simulink model "sampleModel1501"  (R2023a)
settings: Solver=VariableStepAuto  StartTime=0.0  StopTime=10.0  RelTol=1e-3
libraries: hdlsllib x5, simulink x1
settings Model: Creator=user1  LastModifiedBy=user1

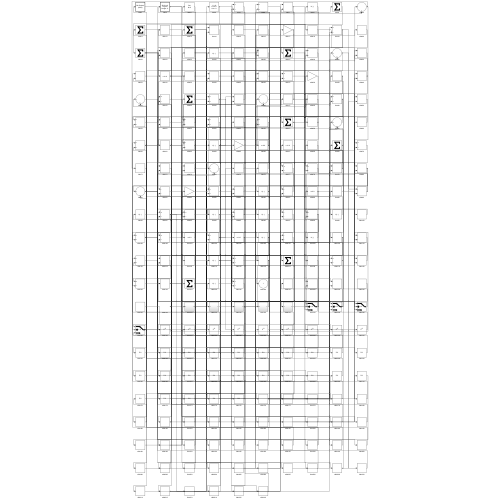
[thumbnail: Simulink's stored preview of the top-level diagram]
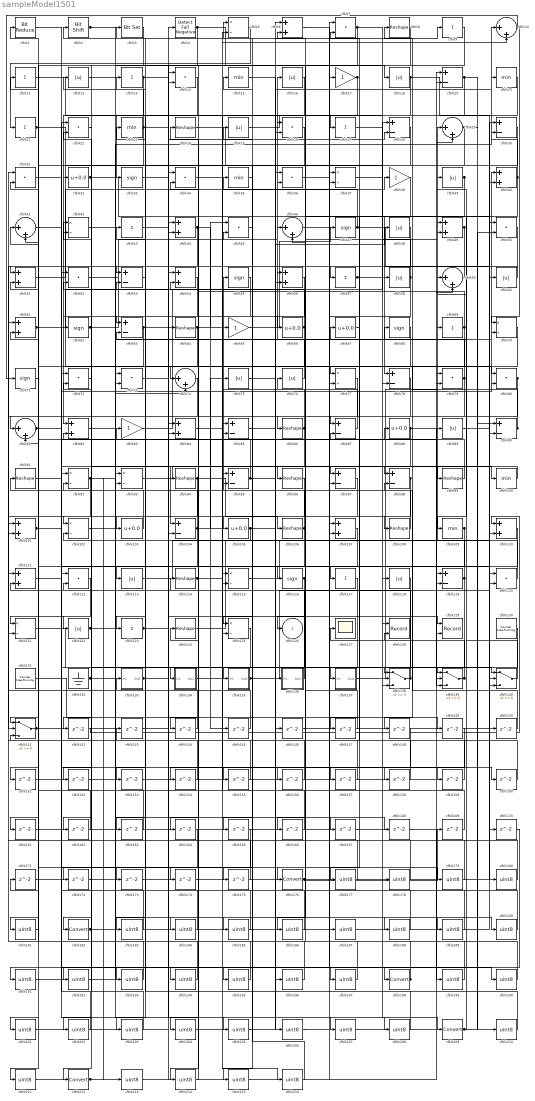
== system sampleModel1501 ==
  cfblk1 : hdlsllib/Logic and Bit Operations/Bit Reduce  mode=AND
  cfblk{10,29,41,46,59,74,81} (7 alike) : Sum  Inputs=|++
  cfblk{15,20,23,35,100,109} (6 alike) : MinMax
  cfblk{6,40,44,49,51,54,56,61,82,84,101,107,110..111} (14 alike) : Sum
  cfblk{5,37,42,70,77,92..93,102,115,121,125} (11 alike) : Product  Inputs=*/  RndMeth=Zero  SaturateOnIntegerOverflow=on
  cfblk{32,66..67,88,103,105} (6 alike) : Bias  Bias=0.0  SaturateOnIntegerOverflow=off
  cfblk{19,28,30,53,63,78,85,87,90,95,97..98,104,119} (14 alike) : Sum  Inputs=+-
  cfblk{8,24,64,86,91,94,96,99,106,108,114,124} (12 alike) : Reshape
  cfblk{9,11,13,21,27,43,57,69,117,123} (10 alike) : Sum  Inputs=+
  cfblk{7,14,22,26,31,34,36,45,50,52,72..73,79..80,112,120} (16 alike) : DotProduct  OutDataTypeStr=Inherit: Inherit via internal rule
  cfblk{12,16,18,25,39,48,58,60,75..76,89,113,118,122} (14 alike) : Abs  SaturateOnIntegerOverflow=off
  cfblk{33,47,55,62,68,71,116} (7 alike) : Signum
  cfblk127 : Scope
  cfblk128 : Record  FileSettingsInternal="{\"entries\":[{\"content\":{\"excelSettings\":{\"content\":{},\"type\":\"Streamout.ExcelSettings\"}},\"type\":\"Streamout.FileSettingStorage\",\"uuid\":\"\"}],\"packageUris\":[\"http:\\/\\/schema.mathworks.com\\/mf0\\/streamout_blocks\\/R2020a\"],\"version\":\"1.0\"}"  Layout=[1 1]  SignalsInternal="{\"entries\":[{\"content\":{\"signals\":[{\"content\":{\"blockPath\":[],\"dimensions\":[1],\"domain\":\"\",\"lineColor\":\"#a2142f\",\"plots\":[1],\"port\":1,\"signalID\":1280,\"signalName\":\"XY Graph:1\"},\"type\":\"RecordBlkView.Signal\",\"uuid\":\"\"},{\"content\":{\"blockPath\":[],\"dimensions\":[1],\"domain\":\"\",\"lineColor\":\"#139fff\",\"plots\":[1],\"port\":2,\"signalID\":1283,\"signalName\":\"XY Graph:2\"},\"type\":\"RecordBlkView.Signal\",\"uuid\":\"\"}]},\"type\":\"RecordBlkView.InputSignals\",\"uuid\":\"\"}],\"packageUris\":[\"http:\\/\\/schema.mathworks.com\\/mf0\\/streamout_blocks\\/R2020a\"],\"version\":\"1.0\"}"  VisualizationBindings="{\"xyplotplugin\":{\"info\":[{\"series\":[{\"bindingParametersList\":[{\"parameter\":\"X-Axis\",\"signalID\":1280,\"signalName\":\"XY Graph:1\"},{\"parameter\":\"Y-Axis\",\"signalID\":1283,\"signalName\":\"XY Graph:2\"}],\"seriesID\":5430}],\"subplotID\":1}]}}"  CompatibilityTag=XY  st=-1
  cfblk129 : Record  FileSettingsInternal="{\"entries\":[{\"content\":{\"excelSettings\":{\"content\":{},\"type\":\"Streamout.ExcelSettings\"}},\"type\":\"Streamout.FileSettingStorage\",\"uuid\":\"\"}],\"packageUris\":[\"http:\\/\\/schema.mathworks.com\\/mf0\\/streamout_blocks\\/R2020a\"],\"version\":\"1.0\"}"  Layout=[1 1]  SignalsInternal="{\"entries\":[{\"content\":{\"signals\":[{\"content\":{\"blockPath\":[],\"dimensions\":[1],\"domain\":\"\",\"lineColor\":\"#a2142f\",\"plots\":[1],\"port\":1,\"signalID\":1288,\"signalName\":\"XY Graph:1\"},\"type\":\"RecordBlkView.Signal\",\"uuid\":\"\"},{\"content\":{\"blockPath\":[],\"dimensions\":[1],\"domain\":\"\",\"lineColor\":\"#139fff\",\"plots\":[1],\"port\":2,\"signalID\":1291,\"signalName\":\"XY Graph:2\"},\"type\":\"RecordBlkView.Signal\",\"uuid\":\"\"}]},\"type\":\"RecordBlkView.InputSignals\",\"uuid\":\"\"}],\"packageUris\":[\"http:\\/\\/schema.mathworks.com\\/mf0\\/streamout_blocks\\/R2020a\"],\"version\":\"1.0\"}"  VisualizationBindings="{\"xyplotplugin\":{\"info\":[{\"series\":[{\"bindingParametersList\":[{\"parameter\":\"X-Axis\",\"signalID\":1288,\"signalName\":\"XY Graph:1\"},{\"parameter\":\"Y-Axis\",\"signalID\":1291,\"signalName\":\"XY Graph:2\"}],\"seriesID\":12827}],\"subplotID\":1}]}}"  CompatibilityTag=XY  st=-1
  cfblk130 : hdlsllib/Sources/Counter Free-Running  NumBits=16  tsamp=-1
  cfblk131 : hdlsllib/Sources/Counter Free-Running  NumBits=16  tsamp=-1
  cfblk132 : Ground
  cfblk133 : Subsystem
      settings: LibrarySourceBlock=|
      | hdlsllib/Ports &
      | Subsystems/Subsystem
  cfblk134 : Subsystem
      settings: LibrarySourceBlock=|
      | hdlsllib/Ports &
      | Subsystems/Subsystem
  cfblk135 : Subsystem
      settings: LibrarySourceBlock=|
      | hdlsllib/Ports &
      | Subsystems/Subsystem
  cfblk136 : Subsystem
      settings: LibrarySourceBlock=|
      | hdlsllib/Ports &
      | Subsystems/Subsystem
  cfblk137 : Subsystem
      settings: LibrarySourceBlock=|
      | hdlsllib/Ports &
      | Subsystems/Subsystem
  cfblk{138..141} (4 alike) : Switch  SaturateOnIntegerOverflow=off  InputSameDT=off
  cfblk{142..175} (34 alike) : Delay  SampleTime=1
  cfblk{17,38,65,83} (4 alike) : Gain
  cfblk{176,182,198,209,212} (5 alike) : DataTypeConversion  SaturateOnIntegerOverflow=off  RndMeth=Floor
  cfblk{177..181,183..197,199..208,210..211,213..216} (36 alike) : DataTypeConversion  OutDataTypeStr=uint8  SaturateOnIntegerOverflow=off  RndMeth=Floor
  cfblk2 : hdlsllib/Logic and Bit Operations/Bit Shift  mode=Shift Left Logical  N=0
  cfblk3 : simulink/Logic and Bit Operations/Bit Set  iBit=0
      settings: LibrarySourceBlock=|
      | hdlsllib/Logic and Bit
      | Operations/Bit Set
  cfblk4 : hdlsllib/Logic and Bit Operations/Detect Fall Negative  vinit=0  OutDataTypeStr=boolean
  cfblk126 : Outport  VectorParamsAs1DForOutWhenUnconnected=off
  wires:
  cfblk96/1 -> cfblk105/1
  cfblk65/1 -> cfblk47/1
  cfblk92/1 -> cfblk85/2, cfblk121/1, cfblk74/2, cfblk213/1
  cfblk13/1 -> cfblk82/1, cfblk129/1, cfblk80/1
  cfblk8/1 -> cfblk134/1(In1)
  cfblk94/1 -> cfblk106/1, cfblk101/2
  cfblk60/1 -> cfblk51/1
  cfblk64/1 -> cfblk103/1, cfblk45/1, cfblk139/3, cfblk10/2
  cfblk106/1 -> cfblk125/1, cfblk11/1, cfblk151/1
  cfblk17/1 -> cfblk95/2, cfblk142/1
  cfblk51/1 -> cfblk38/1
  cfblk76/1 -> cfblk16/1
  cfblk136/1(Out1) -> cfblk91/1
  cfblk79/1 -> cfblk8/1, cfblk23/1, cfblk166/1
  cfblk122/1 -> cfblk188/1, cfblk208/1
  cfblk93/1 -> cfblk100/1
  cfblk46/1 -> cfblk17/1
  cfblk40/1 -> cfblk10/1, cfblk109/1
  cfblk62/1 -> cfblk46/1, cfblk138/1
  cfblk25/1 -> cfblk27/1
  cfblk115/1 -> cfblk29/1
  cfblk39/1 -> cfblk78/1, cfblk97/1
  cfblk6/1 -> cfblk198/1
  cfblk19/1 -> cfblk90/1, cfblk97/2, cfblk183/1
  cfblk30/1 -> cfblk113/1
  cfblk32/1 -> cfblk110/2, cfblk184/1
  cfblk20/1 -> cfblk86/1
  cfblk137/1(Out1) -> cfblk49/1
  cfblk123/1 -> cfblk87/2, cfblk159/1
  cfblk10/1 -> cfblk71/1, cfblk70/1
  cfblk108/1 -> cfblk55/1
  cfblk59/1 -> cfblk57/1
  cfblk5/1 -> cfblk21/1
  cfblk52/1 -> cfblk20/1
  cfblk124/1 -> cfblk30/1
  cfblk21/1 -> cfblk128/1, cfblk136/1(In1), cfblk200/1
  cfblk3/1 -> cfblk32/1
  cfblk90/1 -> cfblk40/1, cfblk68/1
  cfblk97/1 -> cfblk102/1
  cfblk88/1 -> cfblk104/1, cfblk140/3
  cfblk86/1 -> cfblk76/1, cfblk122/1
  cfblk99/1 -> cfblk3/1
  cfblk83/1 -> cfblk28/1
  cfblk66/1 -> cfblk63/1, cfblk42/2, cfblk74/1
  cfblk87/1 -> cfblk65/1
  cfblk100/1 -> cfblk98/1
  cfblk98/1 -> cfblk108/1, cfblk126/1
  cfblk119/1 -> cfblk92/2, cfblk186/1
  cfblk50/1 -> cfblk53/1
  cfblk61/1 -> cfblk56/1, cfblk139/2
  cfblk63/1 -> cfblk81/1, cfblk45/2
  cfblk16/1 -> cfblk33/1
  cfblk38/1 -> cfblk96/1
  cfblk53/1 -> cfblk13/1
  cfblk75/1 -> cfblk9/1
  cfblk141/1 -> cfblk64/1, cfblk205/1
  cfblk22/1 -> cfblk182/1
  cfblk24/1 -> cfblk118/1
  cfblk56/1 -> cfblk66/1
  cfblk114/1 -> cfblk26/1, cfblk168/1
  cfblk55/1 -> cfblk84/2
  cfblk103/1 -> cfblk51/2
  cfblk9/1 -> cfblk116/1
  cfblk11/1 -> cfblk58/1
  cfblk54/1 -> cfblk212/1
  cfblk33/1 -> cfblk4/1
  cfblk80/1 -> cfblk87/1, cfblk121/2
  cfblk47/1 -> cfblk25/1, cfblk90/2
  cfblk130/1 -> cfblk135/1(In1)
  cfblk7/1 -> cfblk99/1, cfblk141/1
  cfblk138/1 -> cfblk128/2, cfblk114/1
  cfblk44/1 -> cfblk141/2, cfblk145/1
  cfblk4/1 -> cfblk78/2, cfblk104/2
  cfblk109/1 -> cfblk125/2, cfblk162/1
  cfblk45/1 -> cfblk5/1
  cfblk134/1(Out1) -> cfblk88/1
  cfblk132/1 -> cfblk82/2, cfblk30/2
  cfblk81/1 -> cfblk115/2, cfblk140/2, cfblk80/2
  cfblk139/1 -> cfblk127/1, cfblk39/1
  cfblk58/1 -> cfblk2/1, cfblk77/2
  cfblk49/1 -> cfblk173/1, cfblk174/1
  cfblk42/1 -> cfblk94/1
  cfblk69/1 -> cfblk24/1, cfblk77/1
  cfblk23/1 -> cfblk12/1, cfblk138/2, cfblk120/2, cfblk181/1
  cfblk105/1 -> cfblk102/2, cfblk70/2
  cfblk133/1(Out1) -> cfblk89/1, cfblk28/2
  cfblk14/1 -> cfblk62/1
  cfblk37/1 -> cfblk209/1
  cfblk140/1 -> cfblk69/1
  cfblk18/1 -> cfblk120/1, cfblk26/2
  cfblk95/1 -> cfblk61/2, cfblk48/1
  cfblk121/1 -> cfblk139/1
  cfblk31/1 -> cfblk176/1
  cfblk116/1 -> cfblk164/1, cfblk165/1
  cfblk2/1 -> cfblk140/1, cfblk18/1
  cfblk29/1 -> cfblk138/3, cfblk210/1
  cfblk101/1 -> cfblk117/1, cfblk157/1
  cfblk91/1 -> cfblk85/1
  cfblk1/1 -> cfblk93/2
  cfblk120/1 -> cfblk34/2
  cfblk135/1(Out1) -> cfblk60/1, cfblk189/1
  cfblk104/1 -> cfblk42/1, cfblk123/1, cfblk75/1, cfblk158/1
  cfblk113/1 -> cfblk19/2
  cfblk57/1 -> cfblk137/1(In1), cfblk49/2
  cfblk102/1 -> cfblk67/1
  cfblk142/1 -> cfblk110/1
  cfblk28/1 -> cfblk144/1
  cfblk144/1 -> cfblk1/1
  cfblk145/1 -> cfblk61/1
  cfblk146/1 -> cfblk50/1
  cfblk67/1 -> cfblk147/1
  cfblk147/1 -> cfblk46/2
  cfblk70/1 -> cfblk148/1
  cfblk85/1 -> cfblk149/1
  cfblk150/1 -> cfblk98/2
  cfblk151/1 -> cfblk19/1
  cfblk125/1 -> cfblk152/1
  cfblk152/1 -> cfblk44/1
  cfblk118/1 -> cfblk153/1
  cfblk153/1 -> cfblk5/2
  cfblk77/1 -> cfblk154/1
  cfblk154/1 -> cfblk63/2
  cfblk26/1 -> cfblk155/1
  cfblk155/1 -> cfblk93/1
  cfblk117/1 -> cfblk156/1
  cfblk156/1 -> cfblk101/1
  cfblk157/1 -> cfblk53/2
  cfblk158/1 -> cfblk7/2
  cfblk159/1 -> cfblk92/1
  cfblk27/1 -> cfblk160/1
  cfblk160/1 -> cfblk115/1
  cfblk71/1 -> cfblk161/1
  cfblk161/1 -> cfblk29/2
  cfblk162/1 -> cfblk81/2
  cfblk68/1 -> cfblk163/1
  cfblk163/1 -> cfblk52/1
  cfblk166/1 -> cfblk95/1
  cfblk12/1 -> cfblk167/1
  cfblk169/1 -> cfblk141/3
  cfblk171/1 -> cfblk119/2
  cfblk74/1 -> cfblk172/1
  cfblk172/1 -> cfblk56/2
  cfblk173/1 -> cfblk14/2
  cfblk174/1 -> cfblk59/2
  cfblk48/1 -> cfblk175/1
  cfblk175/1 -> cfblk84/1
  cfblk176/1 -> cfblk169/1, cfblk40/2, cfblk79/2
  cfblk78/1 -> cfblk177/1
  cfblk177/1 -> cfblk31/1
  cfblk167/1 -> cfblk178/1
  cfblk178/1 -> cfblk31/2
  cfblk41/1 -> cfblk179/1
  cfblk179/1 -> cfblk83/1
  cfblk89/1 -> cfblk180/1
  cfblk180/1 -> cfblk41/1
  cfblk181/1 -> cfblk41/2
  cfblk182/1 -> cfblk150/1, cfblk52/2
  cfblk183/1 -> cfblk22/1
  cfblk184/1 -> cfblk22/2
  cfblk143/1 -> cfblk185/1
  cfblk185/1 -> cfblk72/2
  cfblk186/1 -> cfblk143/1
  cfblk36/1 -> cfblk187/1
  cfblk187/1 -> cfblk170/1
  cfblk188/1 -> cfblk36/1
  cfblk189/1 -> cfblk36/2
  cfblk73/1 -> cfblk190/1
  cfblk190/1 -> cfblk119/1
  cfblk170/1 -> cfblk191/1
  cfblk191/1 -> cfblk73/1
  cfblk72/1 -> cfblk192/1
  cfblk192/1 -> cfblk73/2
  cfblk111/1 -> cfblk193/1
  cfblk193/1 -> cfblk72/1
  cfblk149/1 -> cfblk194/1
  cfblk194/1 -> cfblk111/1
  cfblk82/1 -> cfblk195/1
  cfblk195/1 -> cfblk111/2
  cfblk15/1 -> cfblk196/1
  cfblk196/1 -> cfblk133/1(In1)
  cfblk34/1 -> cfblk197/1
  cfblk197/1 -> cfblk15/1
  cfblk198/1 -> cfblk171/1, cfblk124/1
  cfblk168/1 -> cfblk199/1
  cfblk199/1 -> cfblk6/1
  cfblk200/1 -> cfblk6/2
  cfblk112/1 -> cfblk201/1
  cfblk201/1 -> cfblk14/1
  cfblk110/1 -> cfblk202/1
  cfblk202/1 -> cfblk112/1
  cfblk164/1 -> cfblk203/1
  cfblk203/1 -> cfblk112/2
  cfblk107/1 -> cfblk204/1
  cfblk204/1 -> cfblk146/1
  cfblk205/1 -> cfblk107/1
  cfblk131/1 -> cfblk206/1
  cfblk206/1 -> cfblk107/2
  cfblk43/1 -> cfblk207/1
  cfblk207/1 -> cfblk79/1
  cfblk208/1 -> cfblk43/1
  cfblk209/1 -> cfblk59/1, cfblk50/2
  cfblk210/1 -> cfblk37/1
  cfblk165/1 -> cfblk211/1
  cfblk211/1 -> cfblk37/2
  cfblk212/1 -> cfblk129/2, cfblk44/2, cfblk34/1
  cfblk213/1 -> cfblk54/1
  cfblk148/1 -> cfblk214/1
  cfblk214/1 -> cfblk54/2
  cfblk35/1 -> cfblk215/1
  cfblk215/1 -> cfblk7/1
  cfblk84/1 -> cfblk216/1
  cfblk216/1 -> cfblk35/1

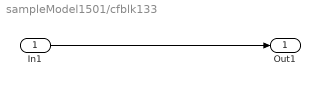
== system sampleModel1501/cfblk133 ==
  In1 : Inport
  Out1 : Outport
  wires:
  In1/1 -> Out1/1

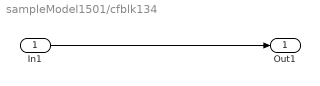
== system sampleModel1501/cfblk134 ==
  In1 : Inport
  Out1 : Outport
  wires:
  In1/1 -> Out1/1

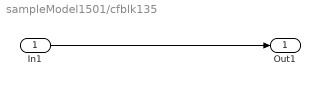
== system sampleModel1501/cfblk135 ==
  In1 : Inport
  Out1 : Outport
  wires:
  In1/1 -> Out1/1

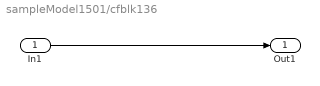
== system sampleModel1501/cfblk136 ==
  In1 : Inport
  Out1 : Outport
  wires:
  In1/1 -> Out1/1

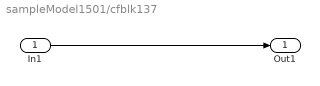
== system sampleModel1501/cfblk137 ==
  In1 : Inport
  Out1 : Outport
  wires:
  In1/1 -> Out1/1
